simulink model "CarrierBasedSVM"  (R2023b)
settings: Solver=FixedStepAuto  StartTime=0.0  StopTime=4/ffund  FixedStep=1e-6  MaxStep=1e-7  RelTol=1e-3
InitFcn:
  | fsw=5500*2;
  | ffund=500;
  | ma=0.5;
libraries: spsTriangleGeneratorLib x2, BoomBox x1, spsdq0toabcLib x1
settings Model: Creator=lbocker  LastModifiedBy=enesa
settings DebuggingCC: SignalInfNanChecking=warning

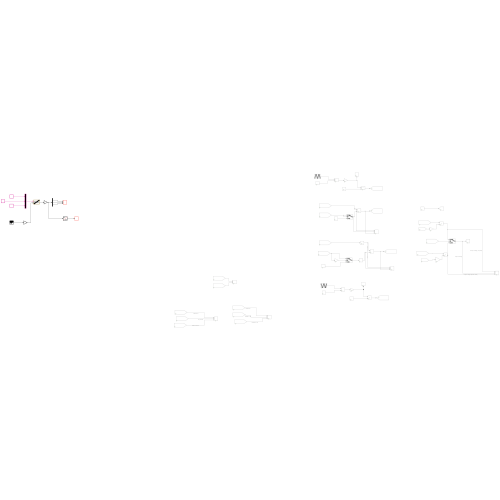
[thumbnail: Simulink's stored preview of the top-level diagram]
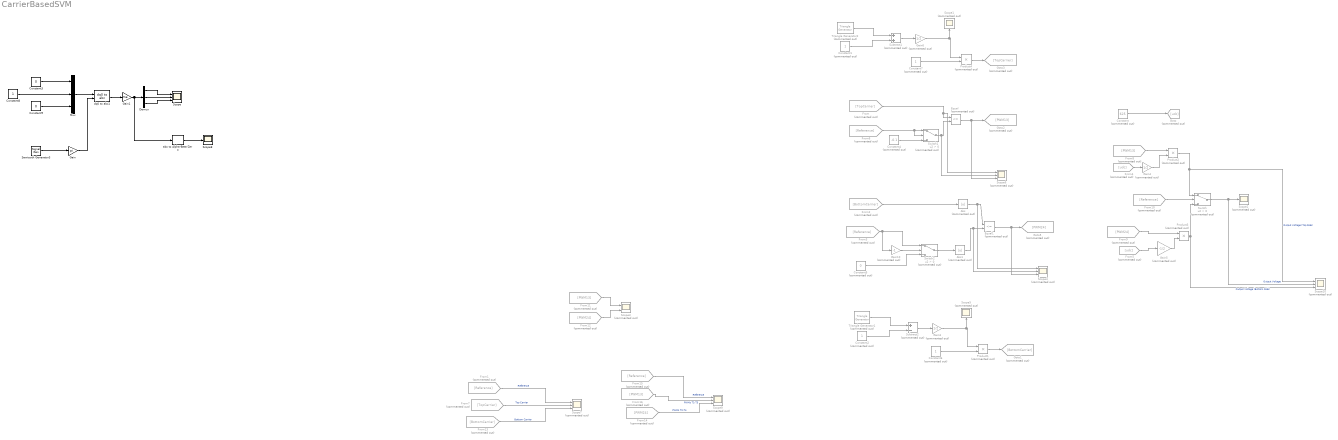
== system CarrierBasedSVM ==
  Abs : Abs  Commented=on  SaturateOnIntegerOverflow=off
  Abs1 : Abs  Commented=on  SaturateOnIntegerOverflow=off
  Constant : Constant  Commented=on  Value=625
  Constant{1..2,6..7} (4 alike) : Constant  Commented=on
  Constant3 : Constant  Value=0
  Constant4 : Constant  Commented=on  Value=-0.1
  Constant5 : Constant  Commented=on  Value=0
  Constant8 : Constant
  Constant9 : Constant  Value=0
  Demux : Demux  Outputs=3
  Equal : RelationalOperator  Commented=on  Operator=<=  OutDataTypeStr=boolean  RndMeth=Simplest  InputSameDT=off
  Equal1 : RelationalOperator  Commented=on  Operator=<=  OutDataTypeStr=boolean  RndMeth=Simplest  InputSameDT=off
  From : From  Commented=on  GotoTag=TopCarrier
  From{1,3,6,10,15} (5 alike) : From  Commented=on  GotoTag=Reference
  From11 : From  Commented=on  GotoTag=PWM13
  From12 : From  Commented=on  GotoTag=PWM24
  From13 : From  Commented=on  GotoTag=BottomCarrier
  From14 : From  Commented=on  GotoTag=PWM24
  From16 : From  Commented=on  GotoTag=PWM13
  From2 : From  Commented=on  GotoTag=BottomCarrier
  From4 : From  Commented=on  GotoTag=udc
  From5 : From  Commented=on  GotoTag=udc
  From7 : From  Commented=on  GotoTag=TopCarrier
  From8 : From  Commented=on  GotoTag=PWM13
  From9 : From  Commented=on  GotoTag=PWM24
  Gain : Gain  Gain=pi
  Gain1 : Gain  Gain=ma
  Gain10 : Gain  Commented=on  Gain=-1
  Gain3 : Gain  Commented=on  Gain=1/2
  Gain4 : Gain  Commented=on  Gain=1/2
  Gain5 : Gain  Commented=on  Gain=-1/2
  Gain6 : Gain  Commented=on  Gain=1/2
  Goto : Goto  Commented=on  GotoTag=udc
  Goto1 : Goto  Commented=on  GotoTag=BottomCarrier
  Goto2 : Goto  Commented=on  GotoTag=PWM13
  Goto3 : Goto  Commented=on  GotoTag=TopCarrier
  Goto5 : Goto  Commented=on  GotoTag=PWM24
  Mux : Mux  Inputs=3
  Product{1..4} (4 alike) : Product  Commented=on
  Sawtooth Generator3 : SignalGenerator  WaveForm=sawtooth  Frequency=2*pi*ffund  Units=rad/sec
  Scope : Scope  NumInputPorts=3
  Scope1 : Scope  Commented=on
  Scope{4,6..7,9..10} (5 alike) : Scope  Commented=on  NumInputPorts=3
  Scope2 : Scope  Commented=on
  Scope3 : Scope  Commented=on  NumInputPorts=2
  Scope5 : Scope  Commented=on
  Scope8 : Scope
  Subtract1 : Sum  Commented=on
  Subtract2 : Sum  Commented=on  Inputs=+-
  Switch : Switch  Commented=on  Criteria=u2 > Threshold  SaturateOnIntegerOverflow=off  InputSameDT=off
  Switch1 : Switch  Commented=on  Criteria=u2 > Threshold  SaturateOnIntegerOverflow=off  InputSameDT=off
  Switch2 : Switch  Commented=on  Criteria=u2 > Threshold  SaturateOnIntegerOverflow=off  InputSameDT=off
  Triangle Generator1 : spsTriangleGeneratorLib/Triangle Generator  Commented=on  Freq=fsw*2  Phase=180  Ts=1e-6
  Triangle Generator2 : spsTriangleGeneratorLib/Triangle Generator  Commented=on  Freq=fsw*2  Phase=0  Ts=1e-6
  abc to Alpha-Beta-Zero : BoomBox/Transformations/abc to Alpha-Beta-Zero  KBID=kb0606
      settings: SourceProductName=imperix blockset
  dq0 to abc1 : spsdq0toabcLib/dq0 to abc  Alignment=90 degrees behind phase A axis
  wires:
  Product3/1 -> Switch/3, Scope10/3  "Output Voltage (Bottom Side)"
  Constant2/1 -> Subtract2/2
  From5/1 -> Gain5/1
  Gain4/1 -> Product2/2
  From4/1 -> Gain4/1
  Gain5/1 -> Product3/2
  Subtract2/1 -> Gain3/1
  Constant6/1 -> Product1/2
  Constant/1 -> Goto/1
  Gain3/1 -> Product1/1, Scope5/1
  Product2/1 -> Scope10/1, Switch/1  "Output Voltage (Top Side)"
  Triangle Generator1/1 -> Subtract2/1
  Switch/1 -> Scope10/2, Scope2/1  "Output Voltage"
  Product1/1 -> Goto1/1
  Product4/1 -> Goto3/1
  Constant7/1 -> Product4/2
  Triangle Generator2/1 -> Subtract1/1
  Constant1/1 -> Subtract1/2
  Gain6/1 -> Product4/1, Scope1/1
  Subtract1/1 -> Gain6/1
  From6/1 -> Switch1/2, Switch1/1
  Constant4/1 -> Switch1/3
  From3/1 -> Gain10/1, Switch2/1
  Switch2/1 -> Abs1/1
  Constant5/1 -> Switch2/3
  Equal/1 -> Scope6/3, Goto2/1
  Equal1/1 -> Scope4/3, Goto5/1
  From8/1 -> Product2/1
  From9/1 -> Product3/1
  From10/1 -> Switch/2
  From11/1 -> Scope3/1
  From12/1 -> Scope3/2
  Gain10/1 -> Switch2/2
  From/1 -> Scope6/1, Equal/1
  Switch1/1 -> Scope6/2, Equal/2
  From1/1 -> Scope7/1  "Reference"
  From7/1 -> Scope7/2  "Top Carrier"
  From13/1 -> Scope7/3  "Bottom Carrier"
  From14/1 -> Scope9/3  "PWMs T2-T4"
  From15/1 -> Scope9/1  "Reference"
  From16/1 -> Scope9/2  "PWMs T1-T3"
  From2/1 -> Abs/1
  Abs/1 -> Scope4/1, Equal1/1
  Abs1/1 -> Scope4/2, Equal1/2
  Sawtooth Generator3/1 -> Gain/1
  dq0 to abc1/1 -> Gain1/1
  Mux/1 -> dq0 to abc1/1
  Constant3/1 -> Mux/1
  Constant8/1 -> Mux/2
  Constant9/1 -> Mux/3
  Demux/1 -> Scope/1
  Demux/2 -> Scope/2
  Demux/3 -> Scope/3
  Gain/1 -> dq0 to abc1/2
  Gain1/1 -> abc to Alpha-Beta-Zero/1, Demux/1
  abc to Alpha-Beta-Zero/1 -> Scope8/1
